simulink library "SingleMotor_V_to_rads"  (R2015a)
settings: Solver=ode45  StartTime=0.0  StopTime=10.0  RelTol=1e-3
undefined symbols (not defined in the file): bm, Jm, Kphi, Lm, Rm, Ubus
libraries: fl_lib x10, nesl_utility x4, SingleMotor_V_to_rads x1
settings Model: Creator=tbaroche  LastModifiedBy=tbaroche

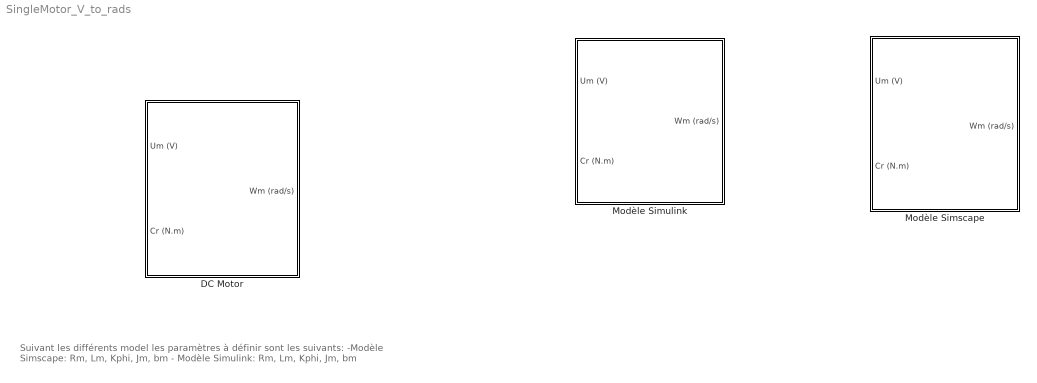
== system SingleMotor_V_to_rads ==
  note: Suivant les différents model les paramètres à définir sont les suivants:
      | 	-Modèle Simscape: Rm, Lm, Kphi, Jm, bm
      | 	- Modèle Simulink: Rm, Lm, Kphi, Jm, bm
  DC Motor : Subsystem  BlockChoice=Modèle Simscape
      settings: TemplateBlock=self  MemberBlocks=Modèle Simscape,Modèle Simulink
  Modèle Simscape : Subsystem  mask{Kphi_lib=Kphi, Rm_lib=Rm, Lm_lib=Lm, bm_lib=bm, Jm_lib=Jm}
      mask prompts: Kphi_lib "Coefficient de couplage:"; Rm_lib "Résistance interne:"; Lm_lib "Inductance propre:"; bm_lib "Coefficient de frottements visqueux:"; Jm_lib "Inertie de l'arbre moteur:"
      mask help: Il s'agit d'un modèle Simscape d'un moteur à courant continu. Ce moteur est commandé en tension. Il est possible de lui applique un couple résistant (Cr).
      mask Display:
      | % A= imread('DCMotor.jpg');
      | % image(A)
      | % port_label('input',1,'Um (V)');
      | % port_label('input',2,'Cr (N.m)');
      | % port_label('output',1,'Wm (rd/s)');
  Modèle Simulink : Subsystem  mask{Kphi_lib=Kphi, Rm_lib=Rm, Lm_lib=Lm, bm_lib=bm, Jm_lib=Jm}
      mask prompts: Kphi_lib "Coefficient de couplage:"; Rm_lib "Résistance interne:"; Lm_lib "Inductance propre:"; bm_lib "Coefficient de frottements visqueux:"; Jm_lib "Inertie de l'arbre moteur:"
      mask help: Il s'agit d'un modèle Simulink d'un moteur à courant continu. Ce moteur est commandé en tension. Il est possible de lui applique un couple résistant (Cr).
      mask Display:
      | % A= imread('DCMotor.jpg');
      | % image(A)
      | % port_label('input',1,'Um (V)');
      | % port_label('input',2,'Cr (N.m)');
      | % port_label('output',1,'Wm (rd/s)');

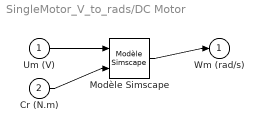
== system SingleMotor_V_to_rads/DC Motor ==
  Um (V) : Inport
  Cr (N.m) : Inport  Port=2
  Modèle Simscape : SingleMotor_V_to_rads/Modèle Simscape  Kphi_lib=Kphi  Rm_lib=Rm  Lm_lib=Lm  bm_lib=bm  Jm_lib=Jm
  Wm (rad/s) : Outport
  wires:
  Um (V)/1 -> Modèle Simscape/1
  Cr (N.m)/1 -> Modèle Simscape/2
  Modèle Simscape/1 -> Wm (rad/s)/1

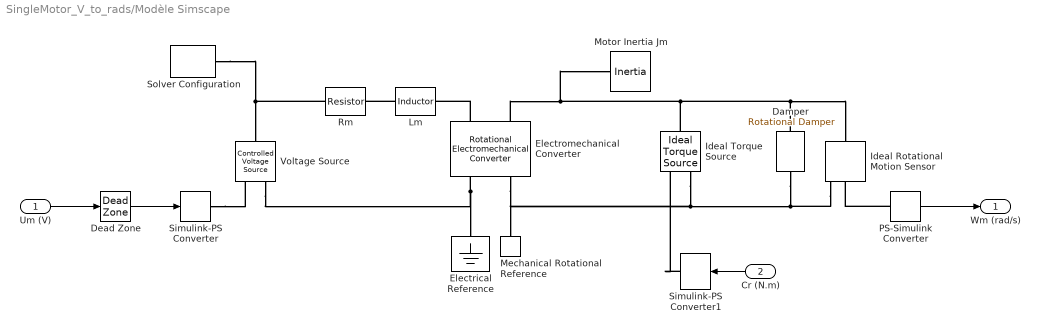
== system SingleMotor_V_to_rads/Modèle Simscape ==
  Um (V) : Inport
  Cr (N.m) : Inport  Port=2
  Damper : fl_lib/Mechanical/Rotational Elements/Rotational Damper  D=bm_lib N*m/(rad/s)  w_specify=off  w_priority=High  w=0 rad/s  t_specify=off  t_priority=High  t=0 N*m
  Dead Zone : DeadZone  LowerValue=-0.22*Ubus  UpperValue=0.22*Ubus  SaturateOnIntegerOverflow=on
  Electrical Reference : fl_lib/Electrical/Electrical Elements/Electrical Reference
  Electromechanical Converter : fl_lib/Electrical/Electrical Elements/Rotational Electromechanical Converter  K=Kphi_lib V/(rad/s)  i_specify=off  i_priority=High  i=0 A  v_specify=off  v_priority=High  v=0 V  t_specify=off  t_priority=High  t=0 N*m  w_specify=off  w_priority=High  w=0 rad/s
  Ideal Torque Source : fl_lib/Mechanical/Mechanical Sources/Ideal Torque Source
  Ideal Rotational Motion Sensor : fl_lib/Mechanical/Mechanical Sensors/Ideal Rotational Motion Sensor  offset=0 rad
  Lm : fl_lib/Electrical/Electrical Elements/Inductor  l=Lm_lib H  r=0 Ohm  g=1e-09 1/Ohm  i_specify=off  i_priority=High  i=0 A  v_specify=off  v_priority=High  v=0 V  i_L_specify=on  i_L_priority=High  i_L=0 A
  Mechanical Rotational Reference : fl_lib/Mechanical/Rotational Elements/Mechanical Rotational Reference
  Motor Inertia Jm : fl_lib/Mechanical/Rotational Elements/Inertia  inertia=Jm_lib kg*m^2  w_specify=on  w_priority=High  w=0 rad/s  t_specify=off  t_priority=High  t=0 N*m
  PS-Simulink Converter : nesl_utility/PS-Simulink Converter  PhysicalDomain=network_engine_domain  SubClassName=ps_output  LeftPortType=input  RightPortType=output  PseudoPeriodic=off  Frequencies=[]  Unit=rad/s  AffineConversion=off
  Rm : fl_lib/Electrical/Electrical Elements/Resistor  Tag=Factory Generic  R=Rm_lib Ohm  i_specify=off  i_priority=High  i=0 A  v_specify=off  v_priority=High  v=0 V
  Simulink-PS Converter : nesl_utility/Simulink-PS Converter  PhysicalDomain=network_engine_domain  SubClassName=ps_input  LeftPortType=input  RightPortType=output  PseudoPeriodic=off  Frequencies=[]  NoiseDistribution=none  NoiseParameters=[]  Unit=V  AffineConversion=off  InputFiltering=off  SimscapeFilterOrder=1  InputFilterTimeConstant=.001  UdotUserProvided=0
  Simulink-PS Converter1 : nesl_utility/Simulink-PS Converter  PhysicalDomain=network_engine_domain  SubClassName=ps_input  LeftPortType=input  RightPortType=output  PseudoPeriodic=off  Frequencies=[]  NoiseDistribution=none  NoiseParameters=[]  Unit=N*m  AffineConversion=off  InputFiltering=off  SimscapeFilterOrder=2  InputFilterTimeConstant=0.001  UdotUserProvided=1
  Solver Configuration : nesl_utility/Solver Configuration  PhysicalDomain=network_engine_domain  SubClassName=solver  LeftPortType=input  RightPortType=generic  Accelerate=off  Tones=[]  Harmonics=[]  SimulateNoise=off  Profile=off  UseLocalSampling=off  EnableSwitchedLinearOptims=on  FrequencyDomain=off  UseCCode=off  RelTol=0.001  AbsTol=1e-06  MinStep=1e-09  ToWorkspace=off  RevertToSquareIcSolve=off  NumHomotopyIterations=100  DoDC=off  ResidualTolerance=1e-9  UseLocalSolver=off  LocalSolverChoice=NE_BACKWARD_EULER_ADVANCER  LocalSolverSampleTime=.001  DoFixedCost=off  MaxNonlinIter=3  MaxModeIter=2  LinearAlgebra=Sparse  DelaysMemoryBudget=1024  AutomaticFiltering=on  FilteringTimeConstant=0.001
  Voltage Source : fl_lib/Electrical/Electrical Sources/Controlled Voltage Source
  Wm (rad/s) : Outport
  wires:
  PS-Simulink Converter/1 -> Wm (rad/s)/1
  Cr (N.m)/1 -> Simulink-PS Converter1/1
  Dead Zone/1 -> Simulink-PS Converter/1
  Um (V)/1 -> Dead Zone/1
  connections:
  Ideal Rotational Motion Sensor/RConn1 -- Electromechanical Converter/RConn2 -- Mechanical Rotational Reference/LConn1 -- Ideal Torque Source/RConn2 -- Damper/RConn1
  Damper/LConn1 -- Ideal Rotational Motion Sensor/LConn1 -- Motor Inertia Jm/LConn1 -- Electromechanical Converter/LConn2 -- Ideal Torque Source/LConn1
  Electromechanical Converter/RConn1 -- Electrical Reference/LConn1 -- Voltage Source/RConn2
  Rm/LConn1 -- Voltage Source/LConn1 -- Solver Configuration/RConn1
  Simulink-PS Converter/RConn1 -- Voltage Source/RConn1
  Electromechanical Converter/LConn1 -- Lm/RConn1
  Lm/LConn1 -- Rm/RConn1
  PS-Simulink Converter/LConn1 -- Ideal Rotational Motion Sensor/RConn2
  Simulink-PS Converter1/RConn1 -- Ideal Torque Source/RConn1

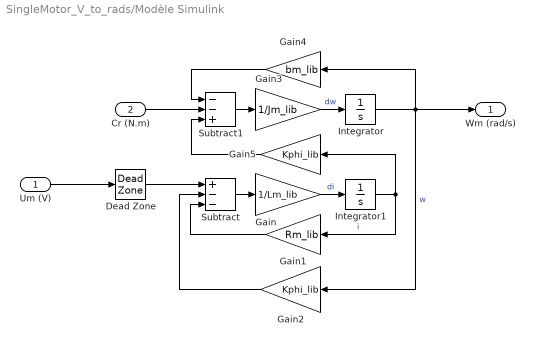
== system SingleMotor_V_to_rads/Modèle Simulink ==
  Um (V) : Inport
  Cr (N.m) : Inport  Port=2
  Dead Zone : DeadZone  LowerValue=-0.22*Ubus  UpperValue=0.22*Ubus  SaturateOnIntegerOverflow=on
  Gain : Gain  Gain=1/Lm_lib
  Gain1 : Gain  Gain=Rm_lib
  Gain2 : Gain  Gain=Kphi_lib
  Gain3 : Gain  Gain=1/Jm_lib
  Gain4 : Gain  Gain=bm_lib
  Gain5 : Gain  Gain=Kphi_lib
  Integrator : Integrator
  Integrator1 : Integrator
  Subtract : Sum  Inputs=+--
  Subtract1 : Sum  Inputs=--+
  Wm (rad/s) : Outport
  wires:
  Gain5/1 -> Subtract1/3
  Gain4/1 -> Subtract1/1
  Subtract/1 -> Gain/1
  Gain1/1 -> Subtract/3
  Integrator1/1 -> Gain5/1, Gain1/1  "i"
  Integrator/1 -> Wm (rad/s)/1, Gain4/1, Gain2/1  "w"
  Gain2/1 -> Subtract/2
  Gain/1 -> Integrator1/1  "di"
  Gain3/1 -> Integrator/1  "dw"
  Cr (N.m)/1 -> Subtract1/2
  Dead Zone/1 -> Subtract/1
  Subtract1/1 -> Gain3/1
  Um (V)/1 -> Dead Zone/1
